simulink model "Modelo_nl111"  (R2015b)
settings: Solver=FixedStepDiscrete  StartTime=20001  StopTime=40000  FixedStep=1  MaxStep=1  RelTol=1e-3
settings Model: Creator=gmiglio  LastModifiedBy=gmiglio

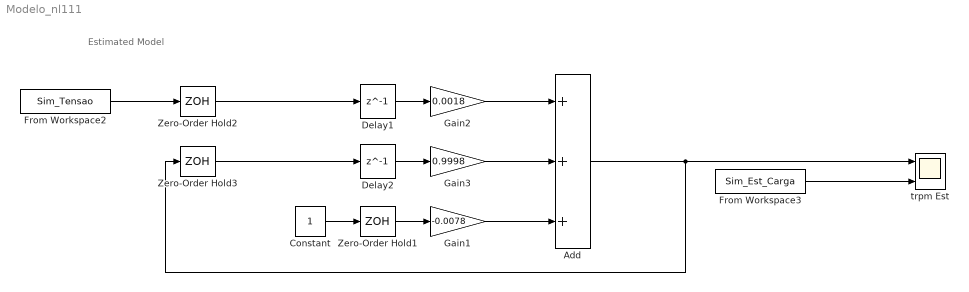
== system Modelo_nl111 ==
  note: Estimated Model
  Add : Sum  Inputs=+++
  Constant : Constant
  Delay1 : Delay  DelayLength=1  InitialCondition=0  SampleTime=1
  Delay2 : Delay  DelayLength=1  InitialCondition=85  SampleTime=1
  From Workspace2 : FromWorkspace  VariableName=Sim_Tensao  SampleTime=0
  From Workspace3 : FromWorkspace  VariableName=Sim_Est_Carga  SampleTime=0
  Gain1 : Gain  Gain=-0.0078
  Gain2 : Gain  Gain=0.0018
  Gain3 : Gain  Gain=0.9998
  Zero-Order Hold1 : ZeroOrderHold
  Zero-Order Hold2 : ZeroOrderHold
  Zero-Order Hold3 : ZeroOrderHold
  trpm Est : Scope  NumInputPorts=2
  wires:
  From Workspace2/1 -> Zero-Order Hold2/1
  Add/1 -> trpm Est/1, Zero-Order Hold3/1
  From Workspace3/1 -> trpm Est/2
  Zero-Order Hold2/1 -> Delay1/1
  Zero-Order Hold3/1 -> Delay2/1
  Delay2/1 -> Gain3/1
  Gain3/1 -> Add/2
  Gain2/1 -> Add/1
  Delay1/1 -> Gain2/1
  Constant/1 -> Zero-Order Hold1/1
  Zero-Order Hold1/1 -> Gain1/1
  Gain1/1 -> Add/3
